simulink model "example12to15"  (R2023b)
settings: Solver=VariableStepAuto  StartTime=0.0  StopTime=10.0  RelTol=1e-3
settings Model: Creator=ray  LastModifiedBy=ray

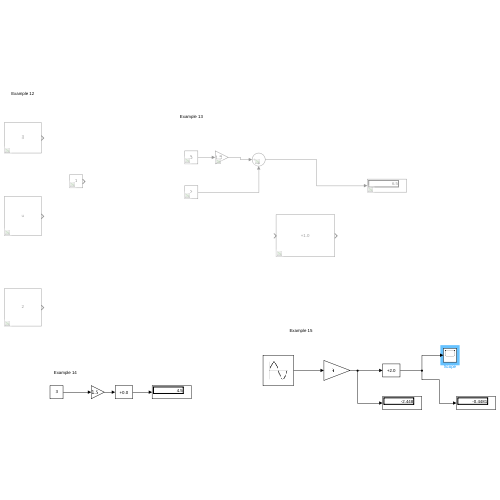
[thumbnail: Simulink's stored preview of the top-level diagram]
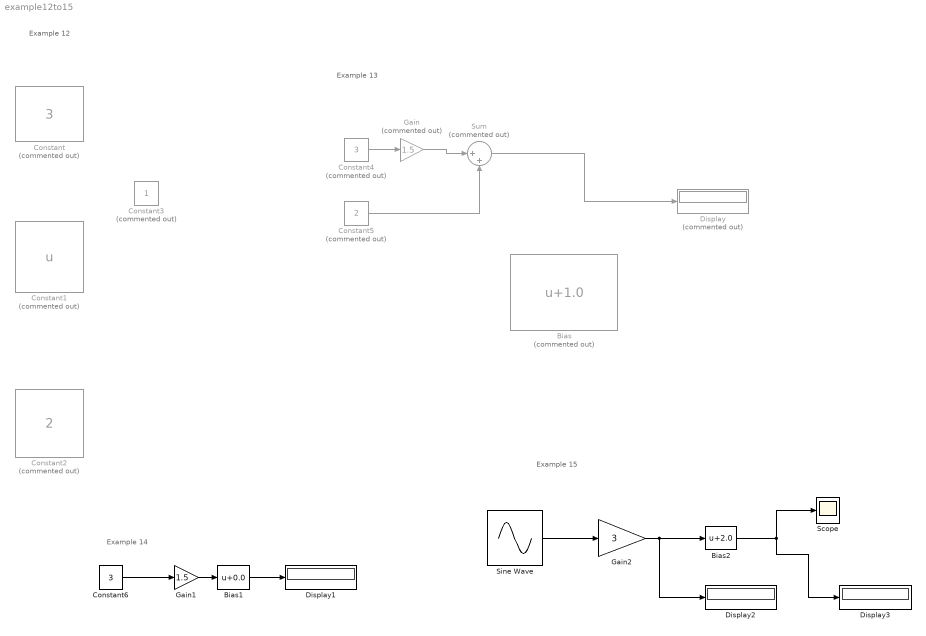
== system example12to15 ==
  note: Example 15
  note: Example 14
  note: Example 13
  note: Example 12
  Bias : Bias  Commented=on  Bias=1.0  SaturateOnIntegerOverflow=off
  Bias1 : Bias  Bias=0.0  SaturateOnIntegerOverflow=off
  Bias2 : Bias  Bias=2.0  SaturateOnIntegerOverflow=off
  Constant : Constant  Commented=on  Value=3
  Constant1 : Constant  Commented=on  Value=u
  Constant2 : Constant  Commented=on  Value=2
  Constant3 : Constant  Commented=on
  Constant4 : Constant  Commented=on  Value=3
  Constant5 : Constant  Commented=on  Value=2
  Constant6 : Constant  Value=3
  Display : Display  Commented=on
  Display1 : Display
  Display2 : Display
  Display3 : Display
  Gain : Gain  Commented=on  Gain=1.5
  Gain1 : Gain  Gain=1.5
  Gain2 : Gain  Gain=3
  Scope : Scope
  Sine Wave : Sin  Amplitude=1.5  SampleTime=0
  Sum : Sum  Commented=on  Inputs=|++
  wires:
  Constant4/1 -> Gain/1
  Gain/1 -> Sum/1
  Constant5/1 -> Sum/2
  Sum/1 -> Display/1
  Constant6/1 -> Gain1/1
  Gain1/1 -> Bias1/1
  Bias1/1 -> Display1/1
  Sine Wave/1 -> Gain2/1
  Gain2/1 -> Display2/1, Bias2/1
  Bias2/1 -> Display3/1, Scope/1
